simulink model "tst_bus_complex_combined_incomplete"  (Simulink 8.0)
settings: Solver=ode45  StartTime=0.0  StopTime=10.0  RelTol=1e-3
settings Model: Creator=Marci  LastModifiedBy=transima

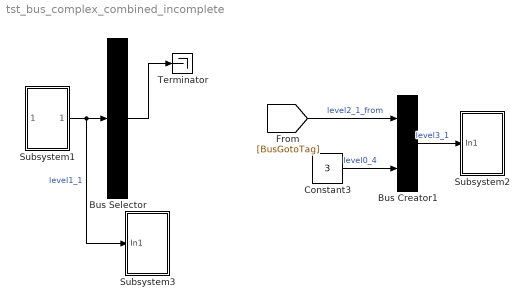
== system tst_bus_complex_combined_incomplete ==
  Bus Creator1 : BusCreator  Inputs=2
  Bus Selector : BusSelector  OutputSignals=level0_1,level0_2  OutputAsBus=on
  Constant3 : Constant  Value=3
  Subsystem1 : Subsystem
  Subsystem2 : Subsystem
  Subsystem3 : Subsystem
  Terminator : Terminator
  wires:
  Bus Selector/1 -> Terminator/1
  Constant3/1 -> Bus Creator1/2  "level0_4"
  Subsystem1/1(Out1) -> Bus Selector/1, Subsystem3/1(In1)  "level1_1"
  Bus Creator1/1 -> Subsystem2/1(In1)  "level3_1"
  [BusGotoTag] -> Bus Creator1/1  "level2_1_from"

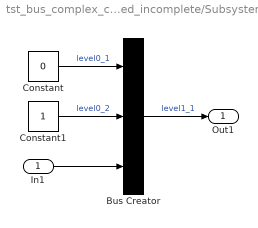
== system tst_bus_complex_combined_incomplete/Subsystem1 ==
  In1 : Inport
  Bus Creator : BusCreator  Inputs=3
  Constant : Constant  Value=0
  Constant1 : Constant
  Out1 : Outport
  wires:
  Constant1/1 -> Bus Creator/2  "level0_2"
  In1/1 -> Bus Creator/3
  Bus Creator/1 -> Out1/1  "level1_1"
  Constant/1 -> Bus Creator/1  "level0_1"

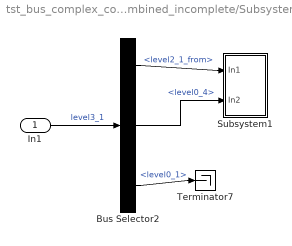
== system tst_bus_complex_combined_incomplete/Subsystem2 ==
  In1 : Inport
  Bus Selector2 : BusSelector  OutputSignals=level2_1_from,level0_4,level2_1_from.level0_1
  Subsystem1 : Subsystem
  Terminator7 : Terminator
  wires:
  Bus Selector2/3 -> Terminator7/1  "<level0_1>"
  In1/1 -> Bus Selector2/1  "level3_1"
  Bus Selector2/1 -> Subsystem1/1(In1)  "<level2_1_from>"
  Bus Selector2/2 -> Subsystem1/2(In2)  "<level0_4>"

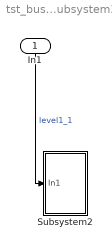
== system tst_bus_complex_combined_incomplete/Subsystem3 ==
  In1 : Inport
  Subsystem2 : Subsystem
  wires:
  In1/1 -> Subsystem2/1(In1)  "level1_1"

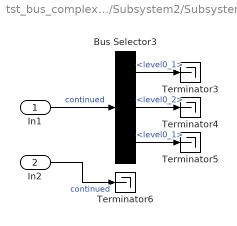
== system tst_bus_complex_combined_incomplete/Subsystem2/Subsystem1 ==
  In1 : Inport
  In2 : Inport  Port=2
  Bus Selector3 : BusSelector  OutputSignals=level0_1,level0_2,level0_1
  Terminator{3..6} (4 alike) : Terminator
  wires:
  Bus Selector3/2 -> Terminator4/1  "<level0_2>"
  Bus Selector3/3 -> Terminator5/1  "<level0_1>"
  In1/1 -> Bus Selector3/1  "continued"
  In2/1 -> Terminator6/1  "continued"
  Bus Selector3/1 -> Terminator3/1  "<level0_1>"

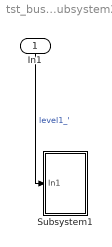
== system tst_bus_complex_combined_incomplete/Subsystem3/Subsystem2 ==
  In1 : Inport
  Subsystem1 : Subsystem
  wires:
  In1/1 -> Subsystem1/1(In1)  "level1_'"

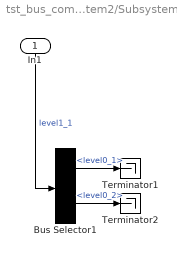
== system tst_bus_complex_combined_incomplete/Subsystem3/Subsystem2/Subsystem1 ==
  In1 : Inport
  Bus Selector1 : BusSelector  OutputSignals=level0_1,level0_2
  Terminator1 : Terminator
  Terminator2 : Terminator
  wires:
  In1/1 -> Bus Selector1/1  "level1_1"
  Bus Selector1/2 -> Terminator2/1  "<level0_2>"
  Bus Selector1/1 -> Terminator1/1  "<level0_1>"
